simulink model "sumiao_github"  (R2019a)
settings: Solver=FixedStepDiscrete  StartTime=0.0  StopTime=totalPixels  FixedStep=1  RelTol=1e-3
InitFcn:
  | frm2pix = visionhdl.FrameToPixels;
  | frm2pix.VideoFormat = '720p';
  | [activePixelsPerLine, activeLines, totalPixels] = getparamfromfrm2pix(frm2pix);
undefined symbols (not defined in the file): gray, Rec, SDTV, totalPixels
libraries: simulink x13, visionhdlio x5, visionhdlutilities x5, visionhdlconversions x1, visionsources x1
settings Model: SimulationMode=accelerator  Creator=linbai  LastModifiedBy=lbai
settings HardwareCC: ProdBitPerPointer=32  ProdBitPerSizeT=32  ProdBitPerPtrDiffT=32  ProdLargestAtomicFloat=None  ProdIntDivRoundTo=Undefined  ProdEndianess=Unspecified  ProdWordSize=32  ProdHWDeviceType=ASIC/FPGA->ASIC/FPGA  TargetBitPerPointer=64  TargetBitPerSizeT=64  TargetBitPerPtrDiffT=64  TargetLongLongMode=on  TargetIntDivRoundTo=Zero  TargetEndianess=LittleEndian  TargetWordSize=64  TargetHWDeviceType=Custom Processor->MATLAB Host Computer  ProdEqTarget=off

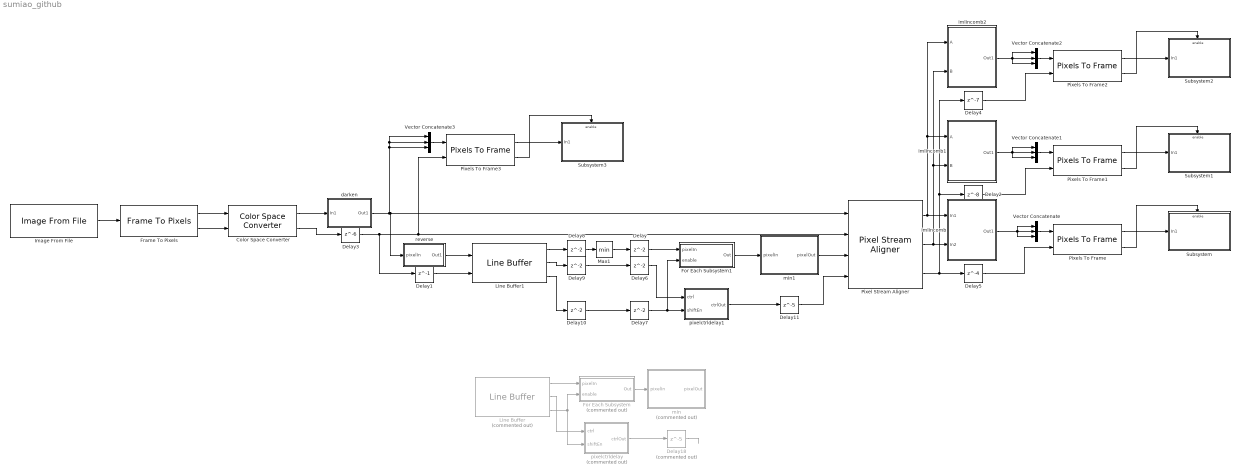
== system sumiao_github ==
  Color Space Converter : visionhdlconversions/Color Space Converter  Conversion=RGB to intensity  ConversionStandard=Rec. 601 (SDTV)  ScanningStandard=1250/50/2:1  SimulateUsing=Code generation
      settings: SourceProductName=Vision HDL Toolbox  SourceProductBaseCode=VT
  Delay{,6..10} (6 alike) : Delay
  Delay1 : Delay  DelayLength=1
  Delay11 : Delay  DelayLength=5
  Delay18 : Delay  Commented=on  DelayLength=5
  Delay2 : Delay  DelayLength=8
  Delay3 : Delay  DelayLength=6
  Delay4 : Delay  DelayLength=7
  Delay5 : Delay  DelayLength=4
  For Each Subsystem : Subsystem  Commented=on  TreatAsAtomicUnit=on
  For Each Subsystem1 : Subsystem  TreatAsAtomicUnit=on
  Frame To Pixels : visionhdlio/Frame To Pixels  NumComponents=3  VideoFormat=720p  ActivePixelsPerLine=160  ActiveVideoLines=160  TotalPixelsPerLine=400  TotalVideoLines=400  StartingActiveLine=6  FrontPorch=120  SampleTime=0
      settings: SourceProductName=Vision HDL Toolbox  SourceProductBaseCode=VT
  Image From File : visionsources/Image From File  Tag=vipblks_nd  FileName=.\sumiao_720p.jpg  Ts=totalPixels  imagePorts=One multidimensional signal  OutPortLabels=R|G|B  ImageDataType=Inherit from input image  sdImageDataType=uint(8)  Signed=on  WordLength=16  FractionLengthMode=User-defined  FractionLength=15
      settings: SourceProductName=Computer Vision Toolbox
  Line Buffer : visionhdlutilities/Line Buffer  Commented=on  NeighborhoodSize=[3 3]  PaddingMethod=Symmetric  PaddingValue=0  LineBufferSize=2048  SimulateUsing=Code generation
      settings: SourceProductName=Vision HDL Toolbox  SourceProductBaseCode=VT
  Line Buffer1 : visionhdlutilities/Line Buffer  NeighborhoodSize=[3 3]  PaddingMethod=Symmetric  PaddingValue=0  LineBufferSize=2048  SimulateUsing=Code generation
      settings: SourceProductName=Vision HDL Toolbox  SourceProductBaseCode=VT
  Max1 : MinMax
  Pixel Stream Aligner : visionhdlutilities/Pixel Stream Aligner  LineBufferSize=2048  MaximumNumberOfLines=10  SimulateUsing=Code generation
      settings: SourceProductName=Vision HDL Toolbox  SourceProductBaseCode=VT
  Pixels To Frame{,1..3} (4 alike) : visionhdlio/Pixels To Frame  NumComponents=3  VideoFormat=720p  ActivePixelsPerLine=160  ActiveVideoLines=160  TotalPixelsPerLine=400  TotalVideoLines=400
      settings: SourceProductName=Vision HDL Toolbox  SourceProductBaseCode=VT
  Subsystem : Subsystem
  Subsystem1 : Subsystem
  Subsystem2 : Subsystem
  Subsystem3 : Subsystem
  Vector Concatenate{,1..3} (4 alike) : Concatenate  NumInputs=3  Mode=Multidimensional array  ConcatenateDimension=2
  darken : Subsystem
  imlincomb : Subsystem
  imlincomb1 : Subsystem
  imlincomb2 : Subsystem
  min : Subsystem  Commented=on
  min1 : Subsystem
  pixelctrldelay : Subsystem  Commented=on
  pixelctrldelay1 : Subsystem
  reverse : Subsystem
  wires:
  Image From File/1 -> Frame To Pixels/1
  Frame To Pixels/1 -> Color Space Converter/1
  Frame To Pixels/2 -> Color Space Converter/2
  Vector Concatenate/1 -> Pixels To Frame/1
  Color Space Converter/2 -> Delay3/1
  Pixels To Frame/1 -> Subsystem/1(In1)
  Pixels To Frame/2 -> Subsystem/Enable
  Color Space Converter/1 -> darken/1(In1)
  Delay1/1 -> Line Buffer1/2
  Pixel Stream Aligner/3 -> Delay5/1, Delay4/1, Delay2/1
  Delay5/1 -> Pixels To Frame/2
  Pixel Stream Aligner/1 -> imlincomb/1(In1), imlincomb2/1(A), imlincomb1/1(A)
  Pixel Stream Aligner/2 -> imlincomb/2(In2), imlincomb2/2(B), imlincomb1/2(B)
  imlincomb1/1(Out1) -> Vector Concatenate1/3, Vector Concatenate1/1, Vector Concatenate1/2
  Delay2/1 -> Pixels To Frame1/2
  Pixels To Frame1/2 -> Subsystem1/Enable
  Pixels To Frame1/1 -> Subsystem1/1(In1)
  Vector Concatenate1/1 -> Pixels To Frame1/1
  imlincomb/1(Out1) -> Vector Concatenate/1, Vector Concatenate/3, Vector Concatenate/2
  Vector Concatenate2/1 -> Pixels To Frame2/1
  Pixels To Frame2/1 -> Subsystem2/1(In1)
  Pixels To Frame2/2 -> Subsystem2/Enable
  Delay4/1 -> Pixels To Frame2/2
  imlincomb2/1(Out1) -> Vector Concatenate2/2, Vector Concatenate2/1, Vector Concatenate2/3
  darken/1(Out1) -> Vector Concatenate3/2, Vector Concatenate3/1, Vector Concatenate3/3, Pixel Stream Aligner/1, reverse/1(pixelIn)
  Delay3/1 -> Pixels To Frame3/2, Pixel Stream Aligner/2, Delay1/1
  Pixels To Frame3/2 -> Subsystem3/Enable
  Pixels To Frame3/1 -> Subsystem3/1(In1)
  Vector Concatenate3/1 -> Pixels To Frame3/1
  Delay7/1 -> For Each Subsystem1/2(enable), pixelctrldelay1/2(shiftEn)
  Delay/1 -> For Each Subsystem1/1(pixelIn)
  Delay6/1 -> pixelctrldelay1/1(ctrl)
  Max1/1 -> Delay/1
  Delay8/1 -> Max1/1
  Line Buffer1/1 -> Delay8/1
  reverse/1(Out1) -> Line Buffer1/1
  Line Buffer1/2 -> Delay9/1
  Delay9/1 -> Delay6/1
  Line Buffer1/3 -> Delay10/1
  Delay10/1 -> Delay7/1
  For Each Subsystem1/1(Out) -> min1/1(pixelIn)
  pixelctrldelay1/1(ctrlOut) -> Delay11/1
  min1/1(pixelOut) -> Pixel Stream Aligner/3
  Delay11/1 -> Pixel Stream Aligner/4
  Delay18/1 -> ?
  Line Buffer/1 -> For Each Subsystem/1(pixelIn)
  Line Buffer/3 -> pixelctrldelay/2(shiftEn), For Each Subsystem/2(enable)
  Line Buffer/2 -> pixelctrldelay/1(ctrl)
  For Each Subsystem/1(Out) -> min/1(pixelIn)
  pixelctrldelay/1(ctrlOut) -> Delay18/1

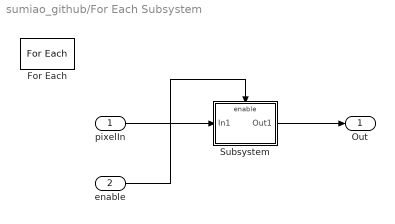
== system sumiao_github/For Each Subsystem ==
  pixelIn : Inport  Partition=on  PartitionDimension=1  PartitionWidth=1  PartitionOffset=0
  enable : Inport  Port=2
  For Each : ForEach  DisableCoverage=on
  Subsystem : Subsystem
  Out : Outport  ConcatenationDimension=1  VectorParamsAs1DForOutWhenUnconnected=on
  wires:
  pixelIn/1 -> Subsystem/1(In1)
  Subsystem/1(Out1) -> Out/1
  enable/1 -> Subsystem/Enable

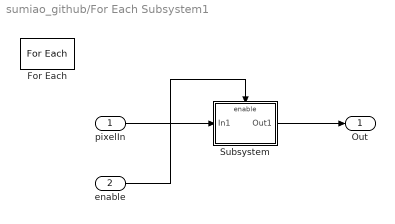
== system sumiao_github/For Each Subsystem1 ==
  pixelIn : Inport  Partition=on  PartitionDimension=1  PartitionWidth=1  PartitionOffset=0
  enable : Inport  Port=2
  For Each : ForEach  DisableCoverage=on
  Subsystem : Subsystem
  Out : Outport  ConcatenationDimension=1  VectorParamsAs1DForOutWhenUnconnected=on
  wires:
  enable/1 -> Subsystem/Enable
  Subsystem/1(Out1) -> Out/1
  pixelIn/1 -> Subsystem/1(In1)

== system sumiao_github/Subsystem ==
  In1 : Inport
  Enable : EnablePort
  Video Viewer : VideoViewer  colormapValue=gray(256)  FigPos=[1922 1011 868 576]
  wires:
  In1/1 -> Video Viewer/1

== system sumiao_github/Subsystem1 ==
  In1 : Inport
  Enable : EnablePort
  Video Viewer : VideoViewer  colormapValue=gray(256)  FigPos=[2717 1013 868 576]
  wires:
  In1/1 -> Video Viewer/1

== system sumiao_github/Subsystem2 ==
  In1 : Inport
  Enable : EnablePort
  Video Viewer : VideoViewer  colormapValue=gray(256)  FigPos=[2034 787 868 576]
  wires:
  In1/1 -> Video Viewer/1

== system sumiao_github/Subsystem3 ==
  In1 : Inport
  Enable : EnablePort
  Video Viewer : VideoViewer  colormapValue=gray(256)  FigPos=[2034 787 868 576]
  wires:
  In1/1 -> Video Viewer/1

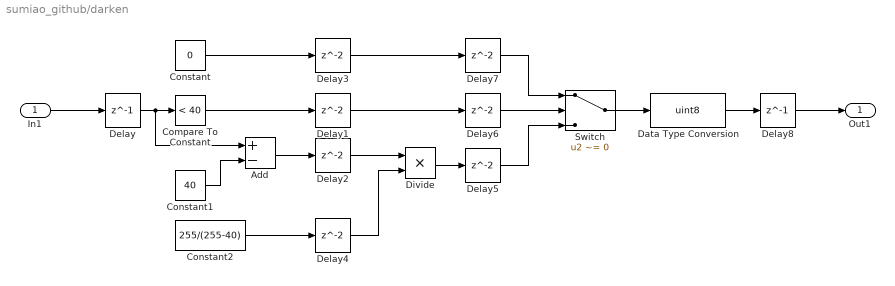
== system sumiao_github/darken ==
  In1 : Inport
  Add : Sum  Inputs=+-
  Compare To Constant : simulink/Logic and Bit Operations/Compare To Constant  relop=<  const=40  OutDataTypeStr=boolean
  Constant : Constant  Value=0  OutDataTypeStr=uint8  SampleTime=-1
  Constant1 : Constant  Value=40  OutDataTypeStr=uint8  SampleTime=-1
  Constant2 : Constant  Value=255/(255-40)  OutDataTypeStr=fixdt(0,16,15)  SampleTime=-1
  Data Type Conversion : DataTypeConversion  OutDataTypeStr=uint8  RndMeth=Round
  Delay : Delay  DelayLength=1
  Delay{1..7} (7 alike) : Delay
  Delay8 : Delay  DelayLength=1
  Divide : Product  Inputs=**
  Switch : Switch  Criteria=u2 ~= 0
  Out1 : Outport  VectorParamsAs1DForOutWhenUnconnected=on
  wires:
  Delay4/1 -> Divide/2
  Delay2/1 -> Divide/1
  Delay6/1 -> Switch/2
  Constant1/1 -> Add/2
  Delay/1 -> Compare To Constant/1, Add/1
  Switch/1 -> Data Type Conversion/1
  Delay1/1 -> Delay6/1
  Constant/1 -> Delay3/1
  Compare To Constant/1 -> Delay1/1
  Divide/1 -> Delay5/1
  Delay7/1 -> Switch/1
  Constant2/1 -> Delay4/1
  Delay5/1 -> Switch/3
  Delay8/1 -> Out1/1
  Delay3/1 -> Delay7/1
  Add/1 -> Delay2/1
  In1/1 -> Delay/1
  Data Type Conversion/1 -> Delay8/1

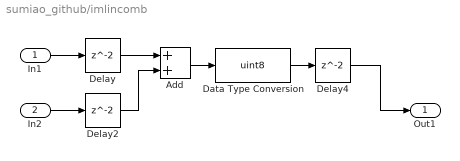
== system sumiao_github/imlincomb ==
  In1 : Inport
  In2 : Inport  Port=2
  Add : Sum
  Data Type Conversion : DataTypeConversion  OutDataTypeStr=uint8
  Delay : Delay
  Delay2 : Delay
  Delay4 : Delay
  Out1 : Outport  VectorParamsAs1DForOutWhenUnconnected=on
  wires:
  Delay4/1 -> Out1/1
  Delay/1 -> Add/1
  Add/1 -> Data Type Conversion/1
  Delay2/1 -> Add/2
  Data Type Conversion/1 -> Delay4/1
  In1/1 -> Delay/1
  In2/1 -> Delay2/1

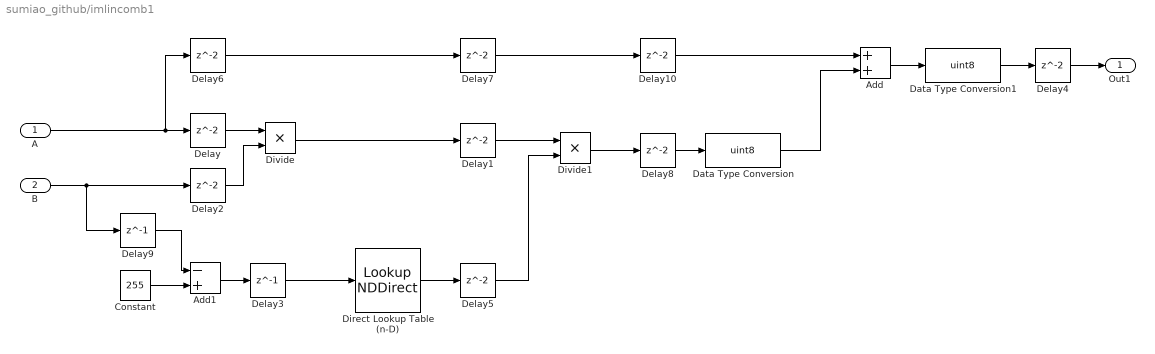
== system sumiao_github/imlincomb1 ==
  A : Inport
  B : Inport  Port=2
  Add : Sum
  Add1 : Sum  Inputs=-+
  Constant : Constant  Value=255  OutDataTypeStr=uint8  SampleTime=-1
  Data Type Conversion : DataTypeConversion  OutDataTypeStr=uint8  SaturateOnIntegerOverflow=on
  Data Type Conversion1 : DataTypeConversion  OutDataTypeStr=uint8  SaturateOnIntegerOverflow=on
  Delay{,1..2,4..8,10} (9 alike) : Delay
  Delay3 : Delay  DelayLength=1
  Delay9 : Delay  DelayLength=1
  Direct Lookup Table (n-D) : LookupNDDirect  NumberOfTableDimensions=1  Table=[0 1./(1:255)]  TableDataTypeStr=fixdt(0,16,15)
  Divide : Product  Inputs=**
  Divide1 : Product  Inputs=**
  Out1 : Outport  VectorParamsAs1DForOutWhenUnconnected=on
  wires:
  B/1 -> Delay9/1, Delay2/1
  A/1 -> Delay6/1, Delay/1
  Delay2/1 -> Divide/2
  Delay8/1 -> Data Type Conversion/1
  Delay/1 -> Divide/1
  Delay4/1 -> Out1/1
  Divide/1 -> Delay1/1
  Delay3/1 -> Direct Lookup Table (n-D)/1
  Direct Lookup Table (n-D)/1 -> Delay5/1
  Delay1/1 -> Divide1/1
  Delay5/1 -> Divide1/2
  Delay6/1 -> Delay7/1
  Divide1/1 -> Delay8/1
  Delay7/1 -> Delay10/1
  Delay10/1 -> Add/1
  Data Type Conversion/1 -> Add/2
  Add/1 -> Data Type Conversion1/1
  Data Type Conversion1/1 -> Delay4/1
  Constant/1 -> Add1/2
  Delay9/1 -> Add1/1
  Add1/1 -> Delay3/1

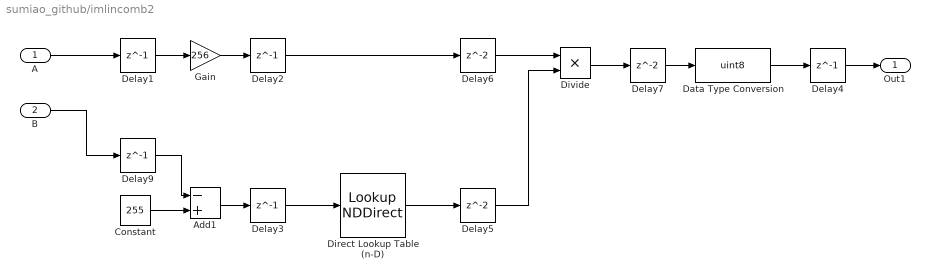
== system sumiao_github/imlincomb2 ==
  A : Inport
  B : Inport  Port=2
  Add1 : Sum  Inputs=-+
  Constant : Constant  Value=255  OutDataTypeStr=uint8  SampleTime=-1
  Data Type Conversion : DataTypeConversion  OutDataTypeStr=uint8  SaturateOnIntegerOverflow=on
  Delay{1..4,9} (5 alike) : Delay  DelayLength=1
  Delay5 : Delay
  Delay6 : Delay
  Delay7 : Delay
  Direct Lookup Table (n-D) : LookupNDDirect  NumberOfTableDimensions=1  Table=[0 1./(1:255)]  TableDataTypeStr=fixdt(0,16,15)
  Divide : Product  Inputs=**
  Gain : Gain  Gain=256
  Out1 : Outport  VectorParamsAs1DForOutWhenUnconnected=on
  wires:
  Add1/1 -> Delay3/1
  Delay9/1 -> Add1/1
  Constant/1 -> Add1/2
  Direct Lookup Table (n-D)/1 -> Delay5/1
  Delay3/1 -> Direct Lookup Table (n-D)/1
  Delay4/1 -> Out1/1
  Delay7/1 -> Data Type Conversion/1
  B/1 -> Delay9/1
  Delay1/1 -> Gain/1
  A/1 -> Delay1/1
  Gain/1 -> Delay2/1
  Delay2/1 -> Delay6/1
  Delay6/1 -> Divide/1
  Delay5/1 -> Divide/2
  Divide/1 -> Delay7/1
  Data Type Conversion/1 -> Delay4/1

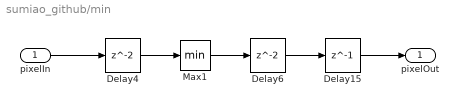
== system sumiao_github/min ==
  pixelIn : Inport
  Delay15 : Delay  DelayLength=1
  Delay4 : Delay
  Delay6 : Delay
  Max1 : MinMax
  pixelOut : Outport  VectorParamsAs1DForOutWhenUnconnected=on
  wires:
  Delay4/1 -> Max1/1
  pixelIn/1 -> Delay4/1
  Max1/1 -> Delay6/1
  Delay15/1 -> pixelOut/1
  Delay6/1 -> Delay15/1

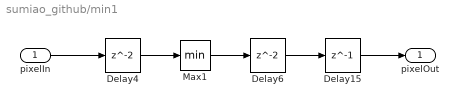
== system sumiao_github/min1 ==
  pixelIn : Inport
  Delay15 : Delay  DelayLength=1
  Delay4 : Delay
  Delay6 : Delay
  Max1 : MinMax
  pixelOut : Outport  VectorParamsAs1DForOutWhenUnconnected=on
  wires:
  Delay6/1 -> Delay15/1
  Delay15/1 -> pixelOut/1
  Max1/1 -> Delay6/1
  pixelIn/1 -> Delay4/1
  Delay4/1 -> Max1/1

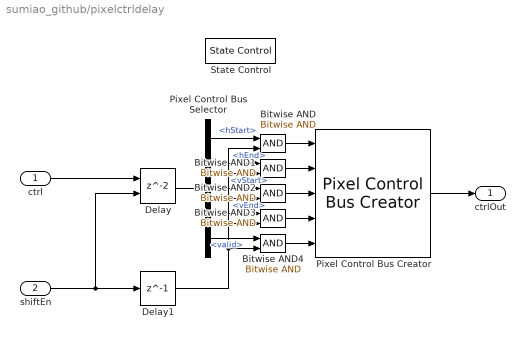
== system sumiao_github/pixelctrldelay ==
  ctrl : Inport
  shiftEn : Inport  Port=2
  Bitwise AND{,1..4} (5 alike) : simulink/Logic and Bit Operations/Bitwise Operator  logicop=AND  UseBitMask=off  NumInputPorts=2  BitMask=bin2dec('11011001')  BitMaskRealWorld=Stored Integer
  Delay : Delay  ShowEnablePort=on
      settings: InputPortMap=u0,e6
  Delay1 : Delay  DelayLength=1
  Pixel Control Bus Creator : visionhdlutilities/Pixel Control Bus Creator
      settings: SourceProductName=Vision HDL Toolbox  SourceProductBaseCode=VT
  Pixel Control Bus Selector : BusSelector  OutputSignals=hStart,hEnd,vStart,vEnd,valid
  State Control : StateControl  StateControl=Synchronous
  ctrlOut : Outport
  wires:
  Bitwise AND4/1 -> Pixel Control Bus Creator/5
  Bitwise AND/1 -> Pixel Control Bus Creator/1
  Pixel Control Bus Selector/3 -> Bitwise AND2/1  "<vStart>"
  Bitwise AND3/1 -> Pixel Control Bus Creator/4
  Pixel Control Bus Selector/5 -> Bitwise AND4/1  "<valid>"
  Delay/1 -> Pixel Control Bus Selector/1
  Pixel Control Bus Selector/1 -> Bitwise AND/1  "<hStart>"
  Pixel Control Bus Selector/2 -> Bitwise AND1/1  "<hEnd>"
  Bitwise AND2/1 -> Pixel Control Bus Creator/3
  Pixel Control Bus Selector/4 -> Bitwise AND3/1  "<vEnd>"
  Bitwise AND1/1 -> Pixel Control Bus Creator/2
  Pixel Control Bus Creator/1 -> ctrlOut/1
  ctrl/1 -> Delay/1
  shiftEn/1 -> Delay1/1, Delay/2
  Delay1/1 -> Bitwise AND3/2, Bitwise AND2/2, Bitwise AND1/2, Bitwise AND/2, Bitwise AND4/2

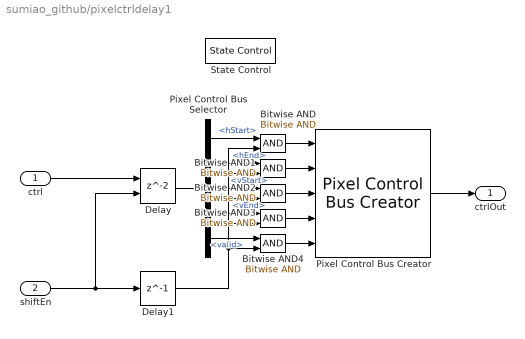
== system sumiao_github/pixelctrldelay1 ==
  ctrl : Inport
  shiftEn : Inport  Port=2
  Bitwise AND{,1..4} (5 alike) : simulink/Logic and Bit Operations/Bitwise Operator  logicop=AND  UseBitMask=off  NumInputPorts=2  BitMask=bin2dec('11011001')  BitMaskRealWorld=Stored Integer
  Delay : Delay  ShowEnablePort=on
      settings: InputPortMap=u0,e6
  Delay1 : Delay  DelayLength=1
  Pixel Control Bus Creator : visionhdlutilities/Pixel Control Bus Creator
      settings: SourceProductName=Vision HDL Toolbox  SourceProductBaseCode=VT
  Pixel Control Bus Selector : BusSelector  OutputSignals=hStart,hEnd,vStart,vEnd,valid
  State Control : StateControl  StateControl=Synchronous
  ctrlOut : Outport
  wires:
  Delay1/1 -> Bitwise AND4/2, Bitwise AND/2, Bitwise AND1/2, Bitwise AND2/2, Bitwise AND3/2
  shiftEn/1 -> Delay/2, Delay1/1
  ctrl/1 -> Delay/1
  Pixel Control Bus Creator/1 -> ctrlOut/1
  Bitwise AND1/1 -> Pixel Control Bus Creator/2
  Pixel Control Bus Selector/4 -> Bitwise AND3/1  "<vEnd>"
  Bitwise AND2/1 -> Pixel Control Bus Creator/3
  Pixel Control Bus Selector/2 -> Bitwise AND1/1  "<hEnd>"
  Pixel Control Bus Selector/1 -> Bitwise AND/1  "<hStart>"
  Delay/1 -> Pixel Control Bus Selector/1
  Pixel Control Bus Selector/5 -> Bitwise AND4/1  "<valid>"
  Bitwise AND3/1 -> Pixel Control Bus Creator/4
  Pixel Control Bus Selector/3 -> Bitwise AND2/1  "<vStart>"
  Bitwise AND/1 -> Pixel Control Bus Creator/1
  Bitwise AND4/1 -> Pixel Control Bus Creator/5

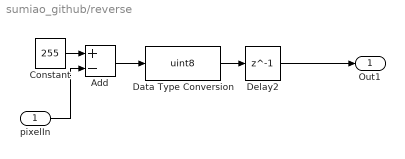
== system sumiao_github/reverse ==
  pixelIn : Inport
  Add : Sum  Inputs=+-
  Constant : Constant  Value=255  OutDataTypeStr=uint8
  Data Type Conversion : DataTypeConversion  OutDataTypeStr=uint8
  Delay2 : Delay  DelayLength=1
  Out1 : Outport  VectorParamsAs1DForOutWhenUnconnected=on
  wires:
  pixelIn/1 -> Add/2
  Constant/1 -> Add/1
  Data Type Conversion/1 -> Delay2/1
  Add/1 -> Data Type Conversion/1
  Delay2/1 -> Out1/1

== system sumiao_github/For Each Subsystem/Subsystem ==
  In1 : Inport
  Enable : EnablePort
  State Control : StateControl  StateControl=Synchronous
  Tapped Delay : simulink/Discrete/Tapped Delay  vinit=0.0  samptime=-1  NumDelays=3  DelayOrder=Oldest  includeCurrent=off
  Out1 : Outport  VectorParamsAs1DForOutWhenUnconnected=on
  wires:
  In1/1 -> Tapped Delay/1
  Tapped Delay/1 -> Out1/1

== system sumiao_github/For Each Subsystem1/Subsystem ==
  In1 : Inport
  Enable : EnablePort
  State Control : StateControl  StateControl=Synchronous
  Tapped Delay : simulink/Discrete/Tapped Delay  vinit=0.0  samptime=-1  NumDelays=3  DelayOrder=Oldest  includeCurrent=off
  Out1 : Outport  VectorParamsAs1DForOutWhenUnconnected=on
  wires:
  Tapped Delay/1 -> Out1/1
  In1/1 -> Tapped Delay/1
